simulink model "twozonevav"  (R2020a)
settings: Solver=FixedStepAuto  StartTime=0.0  StopTime=Inf  FixedStep=0.001  RelTol=1e-3
PostLoadFcn:
  | if any(exist('dsrtsu_mdlpostloadfcn', 'file') ~= 0), dsrtsu_mdlpostloadfcn('Execute', bdroot); end
InitFcn:
  | , if any(exist('rtifpga_mdlclblib', 'file') ~= 0), rtifpga_mdlclblib('Init', bdroot); end,
  | , if any(exist('dsmpb_private', 'file') ~= 0), dsmpb_private('dsmpb_mdlclblib', 'Init', bdroot); end,
libraries: dsmpblib x8
(part 1 of 3)
PreSaveFcn:
  | , if any(exist('dsmpb_private', 'file') ~= 0), dsmpb_private('dsmpb_mdlclblib', 'PreSave', bdroot); end,
CloseFcn:
  | , if any(exist('dsmpb_private', 'file') ~= 0), dsmpb_private('dsmpb_mdlclblib', 'Close', bdroot); end,
settings Model: RTICANMMDATA=struct('GeneralSetupData',struct('modelroot','D:\github\dspace-modelica-example\simulink\twozonevav','generalsettings',struct('filesettings',struct('destfolder',struct('Name','RTICANMM_FILES','Check',1),'buildfolder',struct('Name','.','Check',1),'AbsDestfolder',struct('Name','D:\github\dspace-modelica-example\simulink\twozonevav\RTICANMM_FILES'),'AbsBuildfolder',struct('Name','D:\github\dspace-modelica-example\simulink\twozonevav'))),'options',struct('addpaths',1,'rmpaths',1,'addtrcexclusion',true,'cannavigator',struct('checkmonitoring',0),'show_usrtrc',0,'use_usrtrc',0),'advanced',struct('options',ones(1,100)),'MPSetup',{{}},'RTI',struct('Type','DSRT','Ver','4.3','Date','02-May-2020'),'modelname','twozonevav','block','twozonevav'))  DSRTSU_INTERNAL_RTIFPGA=160  DSMPB_ID_DATA={'100',struct('BlockId','6dd11bb4-ebec-4f08-8ba6-7ddbcbec7d3b','SignalIds',{{'2fb2bb90-4ec6-48ad-8f81-f1d196760c71'}}),'101',struct('BlockId','2ef807c6-571a-44f3-9a64-946af00fb830','SignalIds',{{'b929fcdd-48af-480b-af6b-b2c3ef490cf9'}}),'102',struct('BlockId','fcb8ffc9-48d0-43e3-97e6-63db34e8a87a','SignalIds',{{'7405cf0b-34b8-4d18-b681-bf257a32f1fc'}}),'103',struct('BlockId','44e3c1f1-df5a-4dd4-b5d4-1957fbd80a33','SignalIds',{{'7449a4d7-6efa-496e-ad1d-0eb127210326'}}),'104',struct('BlockId','d3fc6cbc-e5ea-45da-a1ff-e6d33e572c72','SignalIds',{{'ae88789f-7deb-4ded-bc5a-6d8a92166d0d'}}),'97',struct('BlockId','c439f065-e928-4c50-b5e3-14eb295499a2','SignalIds',{{'8fe5f31b-da93-4239-8dda-b4cd2b1e3d5b'}}),'98',struct('BlockId','8b35e11d-29bf-41ba-bcb3-e0861426f11f','SignalIds',{{'ce953cd3-6947-465f-be2f-d959c5a96f49'}}),'99',struct('BlockId','4007e34d-3596-41e8-9571-21578a657730','SignalIds',{{'6190f487-0612-4ce8-bb29-664a6f7d7b4d'}})}  Creator=yangyang.fu  LastModifiedBy=yangyang.fu
settings OptimizationCC: BlockReduction=off  ConditionallyExecuteInputs=off  OptimizeBlockIOStorage=off  BufferReuse=off
settings DebuggingCC: TasksWithSamePriorityMsg=none
settings HardwareCC: ProdBitPerPointer=32  ProdBitPerSizeT=32  ProdBitPerPtrDiffT=32  ProdLargestAtomicInteger=Integer  ProdWordSize=32  ProdLongLongMode=on  ProdHWDeviceType=Custom Processor->Custom
settings ModelReferenceCC: EnableParallelModelReferenceBuilds=on
settings SFSimCC: MATLABDynamicMemAlloc=off
settings RTWCC: Description=dSPACE Run-Time Target (for VEOS on Windows and ConfigurationDesk)  SystemTargetFile=dsrt.tlc  GenCodeOnly=on  MakeCommand=make_dsrt  TemplateMakefile=dsrt_default_tmf  RTWVerbose=off  CustomInclude="\"C:\\Program Files\\Dymola 2021\\Source\""
settings STFCustomTargetCC: TargetLangStandard=C99 (ISO)  ParMdlRefBuildCompliant=on  SystemTargetFile=dsrt.tlc
settings GRTTargetCC: CompOptLevelCompliant=off  ConcurrentExecutionCompliant=off  CombineOutputUpdateFcns=off  MatFileLogging=off  CPPClassGenCompliant=off  UseToolchainInfoCompliant=off

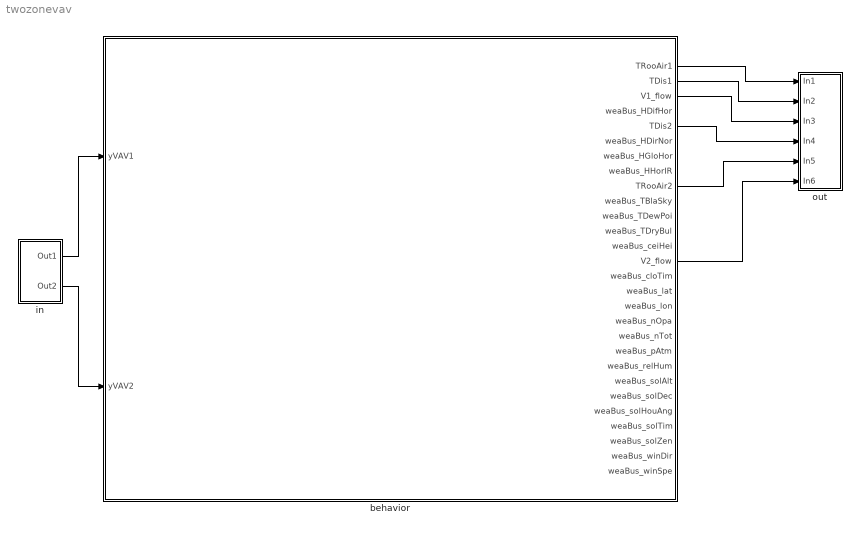
== system twozonevav ==
  behavior : Subsystem
  in : Subsystem
  out : Subsystem
  wires:
  behavior/1(TRooAir1) -> out/1(In1)
  behavior/2(TDis1) -> out/2(In2)
  behavior/3(V1_flow) -> out/3(In3)
  behavior/5(TDis2) -> out/4(In4)
  behavior/9(TRooAir2) -> out/5(In5)
  behavior/14(V2_flow) -> out/6(In6)
  in/1(Out1) -> behavior/1(yVAV1)
  in/2(Out2) -> behavior/2(yVAV2)

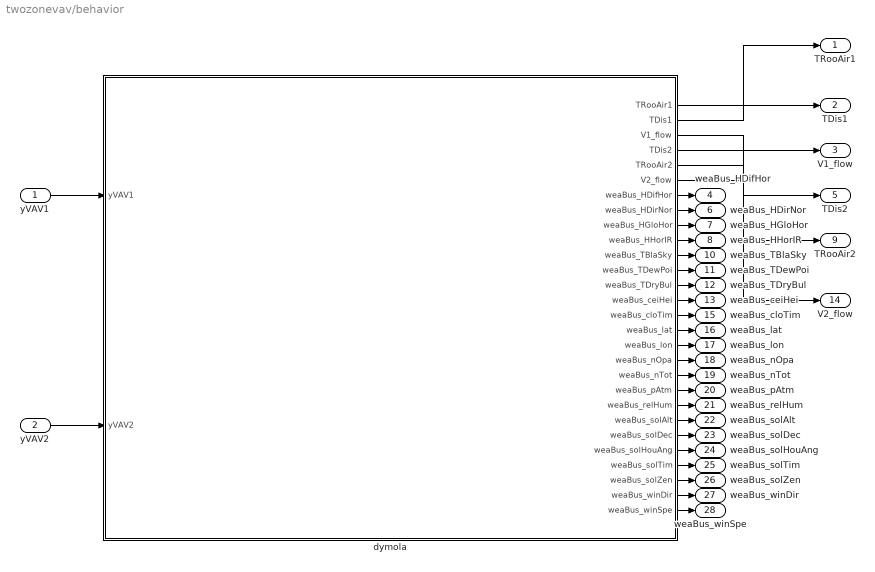
== system twozonevav/behavior ==
  yVAV1 : Inport
  yVAV2 : Inport  Port=2
  dymola : Subsystem  Tag=08-Nov-2021 15:51:38#975
      mask help:
      | Dymola block.
      | A dymola block allows acausal physical modeling.
      | See Dymola manual for usage.
      settings: CopyFcn=newDymolaGui('08-Nov-2021 15:51:38#975','Copy');  DeleteFcn=if exist('newDymolaGui') newDymolaGui('twozonevav/behavior/dymola','Delete'); end;  NameChangeFcn=newDymolaGui('08-Nov-2021 15:51:38#975','Copy');  OpenFcn=newDymolaGui('twozonevav/behavior/dymola','Init');
      mask Display: image(reshape([1;1;1;1;1;1;1;1;1;1;1;1;1;1;1;1;1;1;1;1;1;1;0;0;0;0;0;0;0;0;0;0;1;1;1;1;1;1;1;1;0;1;1;1;1;1;1;1;1;0;1;1;1;1;1;0;0;0;0;0;0;0;1;1;0;0;0;0;0;0;0;1;1;0;0;0;0;0;0;0;1;1;0;0;0;0;0;0;0;1;1;0;0;0;0;0;0;0;1;1;0;0;0;0;0;0;0;1;1;0;0;0;0;0;0;0;1;1;0;0;0;0;0;0;0;1;1;0;0;0;0;0;0;0;1;1;0;0;0;0;0;0;0;1;1;0;0;0;0;0;0;0;1;1;0;0;0;0;0;0;0;1;1;0;0;0;0;0;0;0;1;1;0;0;0;0;0;0;0;1;1;0;0;0;0;0;0;0;1;1;0;0;0;0;0;0;0;1;1;0;0;0;0;0;0;0;1;1;0;0;0;0;0;0;0;1;1;0;0;0;0;0;0;0;1;1;0;0;0;0;0;0;0;1;1;0;0;0;0;0;0;0;1;1;0;0;0;0;0;0;0;1;1;0;0;0;0;0;0;0;1;1;0;0;0;0;0;0;0;1;1;1;1;1;0;1;1;1;1;1;1;1;1;0;1;1;1;1;1;1;1;1;0;0;0;0;0;0;0;0;0;0;1;1;1;1;1;1;1;1;1;1;1;1;1;1;1;1;1;1;1;1;1;1;1;1;1;1;1;1;1;1;1;1;1;1;1;1;1;1;1;1;1;1;1;1;0;0;0;0;0;0;0;0;0;0;1;1;1;1;1;1;1;1;0;1;1;1;1;1;1;1;1;0;1;1;1;1;1;0;0;0;0;0;0;0;1;1;0;0;0;0;0;0;0;1;1;0;0;0;0;0;0;0;1;1;0;0;0;0;0;0;0;1;1;0;0;0;0;0;0;0;1;1;0;0;0;0;0;0;0;1;1;0;0;0;0;0;0;0;1;1;0;0;0;0;0;0;0;1;1;0;0;0;0;0;0;0;1;1;0;0;0;0;0;0;0;1;1;0;0;0;0;0;0;0;1;1;0;0;0;0;0;0;0;1;1;0;0;0;0;0;0;0;1;1;0;0;0;0;0;0;0;1;1;0;0;0;0;0;0;0;1;1;0;0;0;0;0;0;0;1;1;0;0;0;0;0;0;0;1;1;0;0;0;0;0;0;0;1;1;0;0;0;0;0;0;0;1;1;0;0;0;0;0;0;0;1;1;0;0;0;0;0;0;0;1;1;0;0;0;0;0;0;0;1;1;0;0;0;0;0;0;0;1;1;0;0;0;0;0;0;0;1;1;1;1;1;0;1;1;1;1;1;1;1;1;0;1;1;1;1;1;1;1;1;0;0;0;0;0;0;0;0;0;0;1;1;1;1;1;1;1;1;1;1;1;1;1;1;1;1;1;1;1;1;1;1;1;1;1;1;1;1;1;1;1;1;1;1;1;1;1;1;1;1;1;1;1;1;0;0;0;0;0;0;0;0;0;0;1;1;1;1;1;1;1;1;0;1;1;1;1;1;1;1;1;0;1;1;1;1;1;0;0;0;0;0;0;0;1;1;0;0;0;0;0;0;0;1;1;0;1;1;1;1;1;0;1;1;0;1;1;1;1;1;0;1;1;0;1;1;1;1;1;0;1;1;0;1;1;1;1;1;0;1;1;0;1;1;1;1;1;0;1;1;0;1;1;1;1;1;0;1;1;0;1;1;1;1;1;0;1;1;0;1;1;1;1;1;0;1;1;0;1;1;1;1;1;0;1;1;0;1;1;1;1;1;0;1;1;0;1;1;1;1;1;0;1;1;0;1;1;1;1;1;0;1;1;0;1;1;1;1;1;0;1;1;0;1;1;1;1;1;0;1;1;0;1;1;1;1;1;0;1;1;0;1;1;1;1;1;0;1;1;0;1;1;1;1;1;0;1;1;0;1;1;1;1;1;0;1;1;0;1;1;1;1;1;0;1;1;0;1;1;1;1;1;0;1;1;0;0;0;0;0;0;0;1;1;0;0;0;0;0;0;0;1;1;1;1;1;0;1;1;1;1;1;1;1;1;0;1;1;1;1;1;1;1;1;0;0;0;0;0;0;0;0;0;0;1;1;1;1;1;1;1;1;1;1;1;1;1;1;1;1;1;1;1;1;1;1],18,18,3),[.2,.2,.6,.6])
  TRooAir1 : Outport
  TDis1 : Outport  Port=2
  V1_flow : Outport  Port=3
  weaBus_HDifHor : Outport  Port=4
  TDis2 : Outport  Port=5
  weaBus_HDirNor : Outport  Port=6
  weaBus_HGloHor : Outport  Port=7
  weaBus_HHorIR : Outport  Port=8
  TRooAir2 : Outport  Port=9
  weaBus_TBlaSky : Outport  Port=10
  weaBus_TDewPoi : Outport  Port=11
  weaBus_TDryBul : Outport  Port=12
  weaBus_ceiHei : Outport  Port=13
  V2_flow : Outport  Port=14
  weaBus_cloTim : Outport  Port=15
  weaBus_lat : Outport  Port=16
  weaBus_lon : Outport  Port=17
  weaBus_nOpa : Outport  Port=18
  weaBus_nTot : Outport  Port=19
  weaBus_pAtm : Outport  Port=20
  weaBus_relHum : Outport  Port=21
  weaBus_solAlt : Outport  Port=22
  weaBus_solDec : Outport  Port=23
  weaBus_solHouAng : Outport  Port=24
  weaBus_solTim : Outport  Port=25
  weaBus_solZen : Outport  Port=26
  weaBus_winDir : Outport  Port=27
  weaBus_winSpe : Outport  Port=28
  wires:
  dymola/8(weaBus_HDirNor) -> weaBus_HDirNor/1
  dymola/20(weaBus_pAtm) -> weaBus_pAtm/1
  dymola/10(weaBus_HHorIR) -> weaBus_HHorIR/1
  dymola/6(V2_flow) -> V2_flow/1
  dymola/2(TDis1) -> TDis1/1
  dymola/1(TRooAir1) -> TRooAir1/1
  yVAV2/1 -> dymola/2(yVAV2)
  dymola/16(weaBus_lat) -> weaBus_lat/1
  dymola/7(weaBus_HDifHor) -> weaBus_HDifHor/1
  dymola/11(weaBus_TBlaSky) -> weaBus_TBlaSky/1
  dymola/9(weaBus_HGloHor) -> weaBus_HGloHor/1
  dymola/12(weaBus_TDewPoi) -> weaBus_TDewPoi/1
  dymola/13(weaBus_TDryBul) -> weaBus_TDryBul/1
  dymola/14(weaBus_ceiHei) -> weaBus_ceiHei/1
  dymola/24(weaBus_solHouAng) -> weaBus_solHouAng/1
  dymola/15(weaBus_cloTim) -> weaBus_cloTim/1
  dymola/17(weaBus_lon) -> weaBus_lon/1
  dymola/18(weaBus_nOpa) -> weaBus_nOpa/1
  dymola/3(V1_flow) -> V1_flow/1
  dymola/19(weaBus_nTot) -> weaBus_nTot/1
  dymola/27(weaBus_winDir) -> weaBus_winDir/1
  dymola/4(TDis2) -> TDis2/1
  dymola/5(TRooAir2) -> TRooAir2/1
  yVAV1/1 -> dymola/1(yVAV1)
  dymola/23(weaBus_solDec) -> weaBus_solDec/1
  dymola/22(weaBus_solAlt) -> weaBus_solAlt/1
  dymola/21(weaBus_relHum) -> weaBus_relHum/1
  dymola/25(weaBus_solTim) -> weaBus_solTim/1
  dymola/26(weaBus_solZen) -> weaBus_solZen/1
  dymola/28(weaBus_winSpe) -> weaBus_winSpe/1

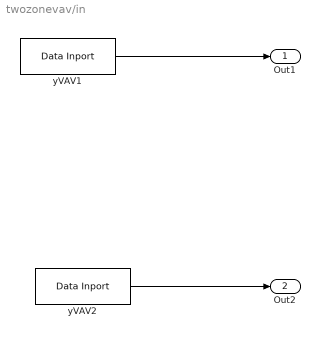
== system twozonevav/in ==
  yVAV1 : dsmpblib/Data Inport  Priority=10000
      settings: SourceProductName=dSPACE Model Interface Blockset
  yVAV2 : dsmpblib/Data Inport  Priority=10000
      settings: SourceProductName=dSPACE Model Interface Blockset
  Out1 : Outport
  Out2 : Outport  Port=2
  wires:
  yVAV1/1 -> Out1/1
  yVAV2/1 -> Out2/1

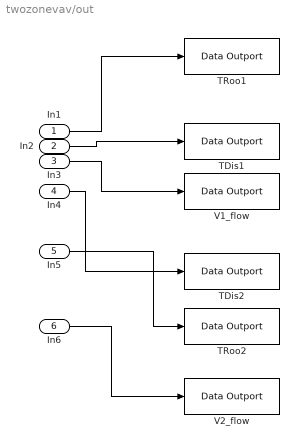
== system twozonevav/out ==
  In1 : Inport
  In2 : Inport  Port=2
  In3 : Inport  Port=3
  In4 : Inport  Port=4
  In5 : Inport  Port=5
  In6 : Inport  Port=6
  TDis1 : dsmpblib/Data Outport  Priority=-10000
      settings: SourceProductName=dSPACE Model Interface Blockset
  TDis2 : dsmpblib/Data Outport  Priority=-10000
      settings: SourceProductName=dSPACE Model Interface Blockset
  TRoo1 : dsmpblib/Data Outport  Priority=-10000
      settings: SourceProductName=dSPACE Model Interface Blockset
  TRoo2 : dsmpblib/Data Outport  Priority=-10000
      settings: SourceProductName=dSPACE Model Interface Blockset
  V1_flow : dsmpblib/Data Outport  Priority=-10000
      settings: SourceProductName=dSPACE Model Interface Blockset
  V2_flow : dsmpblib/Data Outport  Priority=-10000
      settings: SourceProductName=dSPACE Model Interface Blockset
  wires:
  In4/1 -> TDis2/1
  In2/1 -> TDis1/1
  In6/1 -> V2_flow/1
  In5/1 -> TRoo2/1
  In1/1 -> TRoo1/1
  In3/1 -> V1_flow/1
